simulink model "Model_Simulink"  (Simulink 10.3)
settings: Solver=ode3  StartTime=0.0  StopTime=stopTime  FixedStep=0.5  RelTol=1e-3
values from neighbouring files (symbols this model uses):
  OUR = 0.00006    (= 6e-05)    [Model.m]
  So0 = 2.215    [Model.m]
  Sosat = 2.375    [Model.m]
  T0 = 27    [Model.m]
  TkLa = 5    [Model.m]
settings Model: Creator=danie  LastModifiedBy=danie
settings SolverCC: AlgebraicLoopSolver=Auto
settings DataIOCC: SaveFormat=Dataset  SignalLoggingSaveFormat=Dataset  ReturnWorkspaceOutputs=on
settings OptimizationCC: ExpressionDepthLimit=128  LifeSpan=auto
settings DebuggingCC: UnderspecifiedInitializationDetection=Simplified  MergeDetectMultiDrivingBlocksExec=error  FcnCallInpInsideContextMsg=error  StateNameClashWarn=none  SFUnexpectedBacktrackingDiag=error  SFNoUnconditionalDefaultTransitionDiag=error  SFExecutionAtInitializationDiag=warning  SFMachineParentedDataDiag=error  ArithmeticOperatorsInVariantConditions=error
settings HardwareCC: ProdBitPerPointer=64  ProdBitPerSizeT=64  ProdBitPerPtrDiffT=64  ProdLargestAtomicFloat=Float  ProdIntDivRoundTo=Zero  ProdEndianess=LittleEndian  ProdWordSize=64  ProdHWDeviceType=Intel->x86-64 (Windows64)
settings ModelReferenceCC: PropagateSignalLabelsOutOfModel=on
settings SFSimCC: SimUseLocalCustomCode=on  CustomCodeUndefinedFunction=FilterOut
settings RTWCC: RTWUseLocalCustomCode=on
settings CodeAppCC: StateflowObjectComments=off
settings GRTTargetCC: TargetLangStandard=C99 (ISO)  CombineOutputUpdateFcns=on  GRTInterface=off
settings ConfigComp: CovMetricSettings=dwe  CovSaveCumulativeToWorkspaceVar=off  CovSaveSingleToWorkspaceVar=off  CovExternalEMLEnable=on

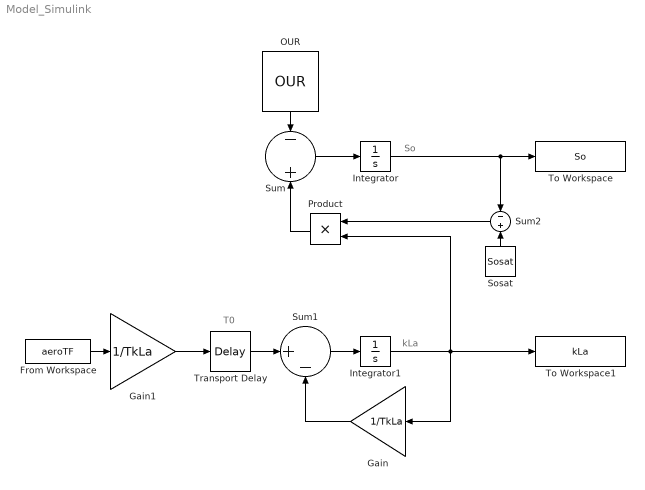
== system Model_Simulink ==
  note: T0
  note: So
  note: kLa
  From Workspace : FromWorkspace  VariableName=aeroTF
  Gain : Gain  Gain=1/TkLa
  Gain1 : Gain  Gain=1/TkLa
  Integrator : Integrator  InitialCondition=So0
  Integrator1 : Integrator
  OUR : Constant  Value=OUR
  Product : Product
  Sosat : Constant  Value=Sosat
  Sum : Sum  Inputs=-+
  Sum1 : Sum  Inputs=|+-
  Sum2 : Sum  Inputs=-|+
  To Workspace : ToWorkspace  VariableName=So  SampleTime=-1
  To Workspace1 : ToWorkspace  VariableName=kLa  SampleTime=-1
  Transport Delay : TransportDelay  DelayTime=T0
  wires:
  Sum1/1 -> Integrator1/1
  Sum/1 -> Integrator/1
  Sosat/1 -> Sum2/2
  Sum2/1 -> Product/1
  Product/1 -> Sum/2
  OUR/1 -> Sum/1
  Integrator/1 -> To Workspace/1, Sum2/1
  Integrator1/1 -> To Workspace1/1, Gain/1, Product/2
  Gain/1 -> Sum1/2
  Transport Delay/1 -> Sum1/1
  Gain1/1 -> Transport Delay/1
  From Workspace/1 -> Gain1/1
